simulink model "salpChain17"  (Simulink 7.8)
settings: Solver=ode15s  StartTime=0.0  StopTime=160  RelTol=1e-3
values from neighbouring files (symbols this model uses):
  angleConstraintB = 25    [15RunsSmallEtta.mat]    (also in 1To10withTorque.mat; 1To20Nodes.mat; 1To30HeadToTail.mat; 1To35FullFlip.mat)
  angleConstraintK = 400    [15RunsSmallEtta.mat]    (also in 1To10withTorque.mat; 1To20Nodes.mat; 1To30HeadToTail.mat; 1To35FullFlip.mat)
  angleLimit = 90    [15RunsSmallEtta.mat]    (also in 1To10withTorque.mat; 1To20Nodes.mat; 1To30HeadToTail.mat; 1To35FullFlip.mat)
  evenTorque = [0 0 0]    [15RunsSmallEtta.mat]    (also in 1To10withTorque.mat = [0 0 0.2]; 1To20Nodes.mat; 1To30HeadToTail.mat; 1To35FullFlip.mat)
  N = size(INPUT,1)    [SpinCalc.m]
  oddTorque = [0 0 0]    [15RunsSmallEtta.mat]    (also in 1To10withTorque.mat = [0 0 0.2]; 1To20Nodes.mat; 1To30HeadToTail.mat; 1To35FullFlip.mat)
  PropSignSw = [-1 -1 1]    [1To10withTorque.mat]    (also in 1To30HeadToTail.mat; 1To35FullFlip.mat)
  relRotInit = [0 0]    [15RunsSmallEtta.mat]    (also in 1To10withTorque.mat; 1To20Nodes.mat; 1To30HeadToTail.mat; 1To35FullFlip.mat)
  sInertia = [0.0008  0  0; 0  0.0008  0; 0  0  0.0004]    [15RunsSmallEtta.mat]    (also in 1To10withTorque.mat; 1To20Nodes.mat; 1To30HeadToTail.mat; 1To35FullFlip.mat)
  sMass = 0.04    [15RunsSmallEtta.mat]    (also in 1To10withTorque.mat; 1To20Nodes.mat; 1To30HeadToTail.mat; 1To35FullFlip.mat)
  uAmplitudeEven = [-1.03766578533 1.19688881264 1.2209450799]    [15RunsSmallEtta.mat]    (also in 1To10withTorque.mat = [-0.2 0 2]; 1To20Nodes.mat = [-0.2 0 2]; 1To30HeadToTail.mat = [-0.2 0 2]; 1To35FullFlip.mat = [-0.2 0.2 2])
libraries: mblibv1 x288
(part 5 of 5)

== system salpChain17/Salp Odd5 ==
  2DOFJointConstrainer : Subsystem
  Body : mblibv1/Bodies/Body  LConnTagsString=CS1  RConnTagsString=CG|CS5|CS4|CS2|CS3|CS6  UpdateFromCAD=off  DialogClass=MechanicalBodyBlock  Mass=sMass  MassUnits=kg  InertiaUnits=kg*m^2  Inertia=sInertia  Shape=Cylinder  ShapeDims=[1 1]  ShapeUnits=m  ShapeUse=false  Density=1  DensityUnits=kg/m^3  DensityUse=false  GraphicsMode=EQELLIPSE  BodyColorSelMode=COLORPALETTE  BodyColor=[0.16471 0.38431 0.27451]  AttachedToCS=CG  CG=Right$CG$frontConnect$CS1$CS1$m$[0 0 0]$Euler X-Y-Z$deg$CS1$true$none  WorkingFrames=Right$CS5$COPPosition$CG$CG$m$[0 0 0]$Euler X-Y-Z$deg$CS1$true$none#Right$CS4$[0 0 0]$CG$CG$m$[0 0 0]$Euler X-Y-Z$deg$CS1$true$none#Left$CS1$[0 0 0]$Adjoining$Adjoining$m$connectR$Euler X-Y-Z$deg$Adjoining$true$none#Right$CS2$backConnect$CG$CG$m$[0 0 0]$Euler X-Y-Z$deg$CS1$true$none#Right$CS3$propulsionPosition$CG$CG$m$[0 0 0]$Euler X-Y-Z$deg$CS1$true$none#Right$CS6$propulsionPosition$CG$CG$m$[0 0 0]$Euler X-Y-Z$deg$CS1$true$none  CGPos=frontConnect  CGRot=[0 0 0]  CS0Pos=[]  CS0Rot=[]  CS1Pos=[0 0 0]  CS1Rot=connectR  CS2Pos=backConnect  CS2Rot=[0 0 0]  CS3Pos=propulsionPosition  CS3Rot=[0 0 0]  CS4Pos=[0 0 0]  CS4Rot=[0 0 0]  CS5Pos=COPPosition  CS5Rot=[0 0 0]  CS6Pos=propulsionPosition  CS6Rot=[0 0 0]  CS7Pos=[]  CS7Rot=[]  CS8Pos=[]  CS8Rot=[]  CS9Pos=[]  CS9Rot=[]  CS10Pos=[]  CS10Rot=[]  CS11Pos=[]  CS11Rot=[]  CS12Pos=[]  CS12Rot=[]  CS13Pos=[]  CS13Rot=[]  CS14Pos=[]  CS14Rot=[]  CS15Pos=[]  CS15Rot=[]  CS16Pos=[]  CS16Rot=[]  CS17Pos=[]  CS17Rot=[]  CS18Pos=[]  CS18Rot=[]  CS19Pos=[]  CS19Rot=[]  CS20Pos=[]  CS20Rot=[]
  Bushing : mblibv1/Joints/Bushing  LConnTagsString=__newl0|SA1  RConnTagsString=__newr0|SA1  UpdateFromCAD=off  NumSAPorts=2  CutJoint=off  MarkAsCut=off  Primitives=prismatic_prismatic_prismatic  PrimitiveProps=P1$Follower$[1 0 0]$prismatic#P2$Follower$[0 1 0]$prismatic#P3$Follower$[0 0 1]$prismatic#R1$Follower$[1 0 0]$revolute#R2$Follower$[0 1 0]$revolute#R3$Follower$[0 0 1]$revolute  DialogClass=JointBlock  P1Axis=[1 0 0]  P2Axis=[0 1 0]  P3Axis=[0 0 1]  R1Axis=[1 0 0]  R2Axis=[0 1 0]  R3Axis=[0 0 1]
  Drag : mblibv1/Sensors &  Actuators/Body Actuator  UpdateFromCAD=off  PhysicalDomain=Mechanical  PortType=blob  ActuationStyle=Force  AngleUnits=deg  ArcVelocityUnits=deg/s  ArcAccelerationUnits=deg/s^2  CoordPositionUnits=m  VelocityUnits=m/s  AccelerationUnits=m/s^2  ForceUnits=N  TorqueUnits=N*m  ActiveIO=off  Width=6  DialogClass=MechanicalActuatorBlock  ReferenceFrame=Local (Body CS)  Angle=off  CoordPosition=on  Force=on  Torque=on
  Force Propulsion : mblibv1/Sensors &  Actuators/Body Actuator  UpdateFromCAD=off  PhysicalDomain=Mechanical  PortType=blob  ActuationStyle=Force  AngleUnits=deg  ArcVelocityUnits=deg/s  ArcAccelerationUnits=deg/s^2  CoordPositionUnits=m  VelocityUnits=m/s  AccelerationUnits=m/s^2  ForceUnits=N  TorqueUnits=N*m  ActiveIO=off  Width=3  DialogClass=MechanicalActuatorBlock  ReferenceFrame=Local (Body CS)  Angle=off  CoordPosition=on  Force=on  Torque=off
  Joint Actuator1 : mblibv1/Sensors &  Actuators/Joint Actuator  UpdateFromCAD=off  PhysicalDomain=Mechanical  PortType=blob  ActuationStyle=Force  AngleUnits=deg  ArcVelocityUnits=deg/s  ArcAccelerationUnits=deg/s^2  CoordPositionUnits=m  VelocityUnits=m/s  AccelerationUnits=m/s^2  ForceUnits=N  TorqueUnits=N*m  ActiveIO=off  Width=1  DialogClass=MechanicalActuatorBlock  Primitive=R1  ReferenceFrame=Absolute (INERTIAL)
  Joint Actuator2 : mblibv1/Sensors &  Actuators/Joint Actuator  UpdateFromCAD=off  PhysicalDomain=Mechanical  PortType=blob  ActuationStyle=Force  AngleUnits=deg  ArcVelocityUnits=deg/s  ArcAccelerationUnits=deg/s^2  CoordPositionUnits=m  VelocityUnits=m/s  AccelerationUnits=m/s^2  ForceUnits=N  TorqueUnits=N*m  ActiveIO=off  Width=1  DialogClass=MechanicalActuatorBlock  Primitive=R2  ReferenceFrame=Absolute (INERTIAL)
  Joint Initial Condition : mblibv1/Sensors &  Actuators/Joint Initial Condition  UpdateFromCAD=off  LeftPortType=blob  RightPortType=blob  PhysicalDomain=mechanical  DialogClass=InitialConditionBlock  InitialConditions=P1$false$0$m$deg$0$m/s$deg/s#P2$false$0$m$deg$0$m/s$deg/s#P3$false$0$m$deg$0$m/s$deg/s#R1$true$relRotInit(1)$m$deg$0$m/s$deg/s#R2$true$relRotInit(2)$m$deg$0$m/s$deg/s#R3$false$0$m$deg$0$m/s$deg/s#S$false$0$m$deg$0$m/s$deg/s  P1PIC=0  P1VIC=0  P2PIC=0  P2VIC=0  P3PIC=0  P3VIC=0  R1PIC=relRotInit(1)  R1VIC=0  R2PIC=relRotInit(2)  R2VIC=0  R3PIC=0  R3VIC=0  SPIC=0  SVIC=0
  Joint Spring & Damper : mblibv1/Force  Elements/Joint Spring & Damper  UpdateFromCAD=off  DialogClass=JointSpringDamper  JFEParameters=P1$true$kDrag(1)$bDrag(1)$0$m$m/s$N$deg$deg/s$N*m#P2$true$kDrag(2)$bDrag(2)$0$m$m/s$N$deg$deg/s$N*m#P3$true$kDrag(3)$bDrag(3)$0$m$m/s$N$deg$deg/s$N*m#R1$true$kDrag(4)$bDrag(4)$0$m$m/s$N$deg$deg/s$N*m#R2$true$kDrag(5)$bDrag(5)$0$m$m/s$N$deg$deg/s$N*m#R3$true$kDrag(6)$bDrag(6)$0$m$m/s$N$deg$deg/s$N*m#S$false$0$0$0$m$m/s$N$deg$deg/s$N*m
  Mechanical Branching Bar : mblibv1/Utilities/Mechanical Branching Bar  LConnTagsString=_newl0  RConnTagsString=__newr0|SA2  UpdateFromCAD=off  DialogClass=MechanicalBranchingBarBlock  NumSAPorts=2
  Mechanical Branching Bar1 : mblibv1/Utilities/Mechanical Branching Bar  LConnTagsString=_newl0  RConnTagsString=__newr0|SA2  UpdateFromCAD=off  DialogClass=MechanicalBranchingBarBlock  NumSAPorts=2
  Model : ModelReference  ModelNameDialog=v2Drag  SimulationMode=Normal  ModelReferenceVersion=1.20  CopyOfModelName=v2Drag  DefaultDataLogging=on
  Mux : Mux  Inputs=2
  Torque Propulsion : mblibv1/Sensors &  Actuators/Body Actuator  UpdateFromCAD=off  PhysicalDomain=Mechanical  PortType=blob  ActuationStyle=Force  AngleUnits=deg  ArcVelocityUnits=deg/s  ArcAccelerationUnits=deg/s^2  CoordPositionUnits=m  VelocityUnits=m/s  AccelerationUnits=m/s^2  ForceUnits=N  TorqueUnits=N*m  ActiveIO=off  Width=3  DialogClass=MechanicalActuatorBlock  ReferenceFrame=Local (Body CS)  Angle=off  CoordPosition=on  Force=off  Torque=on
  Universal : mblibv1/Joints/Universal  LConnTagsString=__newl0|SA1|SA2  RConnTagsString=__newr0|SA1|SA2  UpdateFromCAD=off  NumSAPorts=4  CutJoint=off  MarkAsCut=off  Primitives=prismatic  PrimitiveProps=R1$Base$u1axis$revolute#R2$Base$u2axis$revolute  DialogClass=JointBlock  R1Axis=u1axis  R2Axis=u2axis
  angle 2 : mblibv1/Sensors &  Actuators/Joint Sensor  UpdateFromCAD=off  PhysicalDomain=Mechanical  PortType=blob  Muxed=on  Pose=off  Angle=on  AngleUnits=deg  ArcVelocity=off  ArcVelocityUnits=deg/s  ArcAcceleration=off  ArcAccelerationUnits=deg/s^2  CoordPosition=on  CoordPositionUnits=m  Velocity=off  VelocityUnits=m/s  Acceleration=off  AccelerationUnits=m/s^2  Quaternion=on  QuaternionDT=off  QuaternionDDT=off  QuaternionUnits=off  OutputVector=[1]  ActiveIO=off  Width=1  DialogClass=MechanicalSensorBlock  Primitive=R2  Force=off  ForceUnits=N  Torque=off  TorqueUnits=N*m  ReferenceFrame=Absolute (World)  ReactionSensedSide=Base  ReactionReferenceFrame=Absolute (World)  ReactionForce=off  ReactionForceUnits=N  ReactionMoment=off  ReactionMomentUnits=N*m
  angle1 : mblibv1/Sensors &  Actuators/Joint Sensor  UpdateFromCAD=off  PhysicalDomain=Mechanical  PortType=blob  Muxed=on  Pose=off  Angle=on  AngleUnits=deg  ArcVelocity=off  ArcVelocityUnits=deg/s  ArcAcceleration=off  ArcAccelerationUnits=deg/s^2  CoordPosition=on  CoordPositionUnits=m  Velocity=off  VelocityUnits=m/s  Acceleration=off  AccelerationUnits=m/s^2  Quaternion=on  QuaternionDT=off  QuaternionDDT=off  QuaternionUnits=off  OutputVector=[1]  ActiveIO=off  Width=1  DialogClass=MechanicalSensorBlock  Primitive=R1  Force=off  ForceUnits=N  Torque=off  TorqueUnits=N*m  ReferenceFrame=Absolute (World)  ReactionSensedSide=Base  ReactionReferenceFrame=Absolute (World)  ReactionForce=off  ReactionForceUnits=N  ReactionMoment=off  ReactionMomentUnits=N*m
  angular velocity body frame : mblibv1/Sensors &  Actuators/Body Sensor  UpdateFromCAD=off  PhysicalDomain=Mechanical  PortType=blob  Muxed=off  Pose=off  Angle=on  AngleUnits=deg  ArcVelocity=on  ArcVelocityUnits=deg/s  ArcAcceleration=off  ArcAccelerationUnits=deg/s^2  CoordPosition=off  CoordPositionUnits=m  Velocity=off  VelocityUnits=m/s  Acceleration=off  AccelerationUnits=m/s^2  Quaternion=on  QuaternionDT=off  QuaternionDDT=off  QuaternionUnits=off  OutputVector=[1]  ActiveIO=off  Width=3  DialogClass=MechanicalSensorBlock  ReferenceFrame=Local (Body CS)
  dummy body for drag : mblibv1/Bodies/Body  LConnTagsString=CS1  RConnTagsString=CS2  UpdateFromCAD=off  DialogClass=MechanicalBodyBlock  Mass=sMass/100  MassUnits=kg  InertiaUnits=kg*m^2  Inertia=eye(3)/1000  Shape=Cylinder  ShapeDims=[1 1]  ShapeUnits=m  ShapeUse=false  Density=1  DensityUnits=kg/m^3  DensityUse=false  GraphicsMode=CONVHULL  BodyColorSelMode=COLORPALETTE  BodyColor=[1 0 1]  AttachedToCS=CG  CG=Left$CG$[0 0 0]$CS1$CS1$m$[0 0 0]$Euler X-Y-Z$deg$CS1$false$none  WorkingFrames=Left$CS1$[0 0 0]$Adjoining$Adjoining$m$[0 0 0]$Euler X-Y-Z$deg$Adjoining$true$none#Right$CS2$[0 0 0]$CS1$CS1$m$[0 0 0]$Euler X-Y-Z$deg$CS1$true$none  CGPos=[0 0 0]  CGRot=[0 0 0]  CS0Pos=[]  CS0Rot=[]  CS1Pos=[0 0 0]  CS1Rot=[0 0 0]  CS2Pos=[0 0 0]  CS2Rot=[0 0 0]  CS3Pos=[]  CS3Rot=[]  CS4Pos=[]  CS4Rot=[]  CS5Pos=[]  CS5Rot=[]  CS6Pos=[]  CS6Rot=[]  CS7Pos=[]  CS7Rot=[]  CS8Pos=[]  CS8Rot=[]  CS9Pos=[]  CS9Rot=[]  CS10Pos=[]  CS10Rot=[]  CS11Pos=[]  CS11Rot=[]  CS12Pos=[]  CS12Rot=[]  CS13Pos=[]  CS13Rot=[]  CS14Pos=[]  CS14Rot=[]  CS15Pos=[]  CS15Rot=[]  CS16Pos=[]  CS16Rot=[]  CS17Pos=[]  CS17Rot=[]  CS18Pos=[]  CS18Rot=[]  CS19Pos=[]  CS19Rot=[]  CS20Pos=[]  CS20Rot=[]
  translation body frame : mblibv1/Sensors &  Actuators/Body Sensor  UpdateFromCAD=off  PhysicalDomain=Mechanical  PortType=blob  Muxed=off  Pose=off  Angle=on  AngleUnits=deg  ArcVelocity=off  ArcVelocityUnits=deg/s  ArcAcceleration=off  ArcAccelerationUnits=deg/s^2  CoordPosition=off  CoordPositionUnits=m  Velocity=on  VelocityUnits=m/s  Acceleration=off  AccelerationUnits=m/s^2  Quaternion=on  QuaternionDT=off  QuaternionDDT=off  QuaternionUnits=off  OutputVector=[1]  ActiveIO=off  Width=3  DialogClass=MechanicalSensorBlock  ReferenceFrame=Local (Body CS)
  Front : PMIOPort  Port=1  Side=Left
  Back : PMIOPort  Port=2  Side=Right
  wires:
  translation body frame/1 -> Model/1
  Mux/1 -> Drag/1
  angular velocity body frame/1 -> Model/2
  angle 2/1 -> 2DOFJointConstrainer/2(In2)  "angle2"
  angle1/1 -> 2DOFJointConstrainer/1(In1)  "angle1"
  Model/1 -> Mux/1
  Model/2 -> Mux/2
  [OddAmplitude] -> Force Propulsion/1
  [OddTorque] -> Torque Propulsion/1
  2DOFJointConstrainer/1(Out1) -> Joint Actuator1/1
  2DOFJointConstrainer/2(Out2) -> Joint Actuator2/1
  connections:
  Body/RConn3 -- Mechanical Branching Bar/LConn1
  dummy body for drag/RConn1 -- Drag/RConn1
  Mechanical Branching Bar/RConn1 -- angular velocity body frame/LConn1
  translation body frame/LConn1 -- Mechanical Branching Bar/RConn2
  Bushing/RConn1 -- Body/RConn2
  Bushing/LConn1 -- dummy body for drag/LConn1
  Bushing/RConn2 -- Joint Spring & Damper/LConn1
  Front/RConn1 -- Body/LConn1
  Universal/RConn1 -- Back/RConn1
  Universal/LConn1 -- Body/RConn4
  Universal/LConn2 -- Joint Initial Condition/RConn1
  Force Propulsion/RConn1 -- Body/RConn5
  Universal/RConn2 -- Mechanical Branching Bar1/LConn1
  Mechanical Branching Bar1/RConn1 -- angle1/LConn1
  Mechanical Branching Bar1/RConn2 -- angle 2/LConn1
  Torque Propulsion/RConn1 -- Body/RConn6
  Universal/RConn3 -- Joint Actuator1/RConn1
  Joint Actuator2/RConn1 -- Universal/LConn3

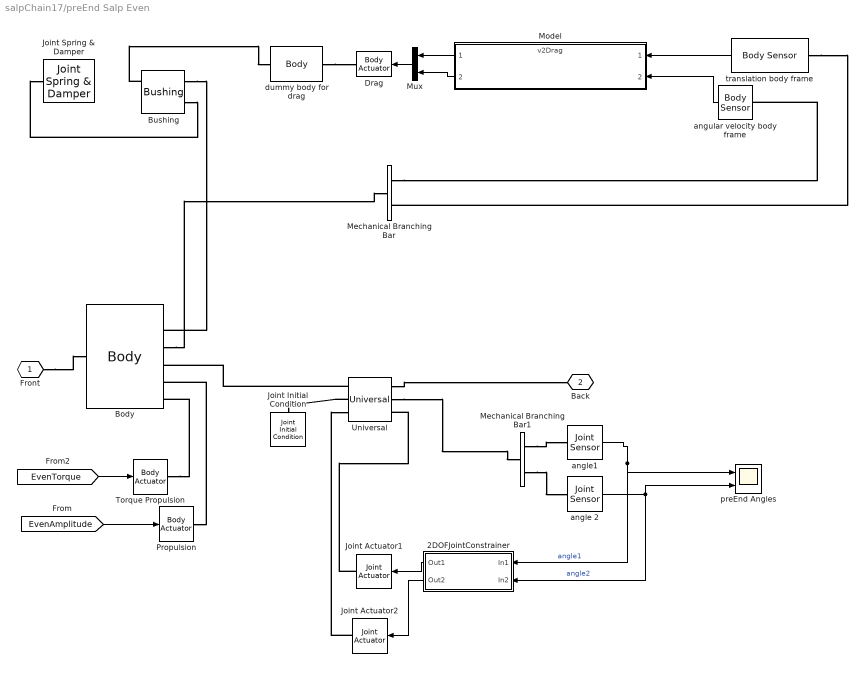
== system salpChain17/preEnd Salp Even ==
  2DOFJointConstrainer : Subsystem
  Body : mblibv1/Bodies/Body  LConnTagsString=CS1  RConnTagsString=CG|CS5|CS4|CS2|CS3|CS6  UpdateFromCAD=off  DialogClass=MechanicalBodyBlock  Mass=sMass  MassUnits=kg  InertiaUnits=kg*m^2  Inertia=sInertia  Shape=Cylinder  ShapeDims=[1 1]  ShapeUnits=m  ShapeUse=false  Density=1  DensityUnits=kg/m^3  DensityUse=false  GraphicsMode=EQELLIPSE  BodyColorSelMode=COLORPALETTE  BodyColor=[0.16471 0.38431 0.27451]  AttachedToCS=CG  CG=Right$CG$frontConnect$CS1$CS1$m$[0 0 0]$Euler X-Y-Z$deg$CS1$true$none  WorkingFrames=Right$CS5$COPPosition$CG$CG$m$[0 0 0]$Euler X-Y-Z$deg$CS1$true$none#Right$CS4$[0 0 0]$CG$CG$m$[0 0 0]$Euler X-Y-Z$deg$CS1$true$none#Left$CS1$[0 0 0]$Adjoining$Adjoining$m$connectR$Euler X-Y-Z$deg$Adjoining$true$none#Right$CS2$backConnect$CG$CG$m$[0 0 0]$Euler X-Y-Z$deg$CS1$true$none#Right$CS3$propulsionPosition$CG$CG$m$[0 0 0]$Euler X-Y-Z$deg$CS1$true$none#Right$CS6$propulsionPosition$CG$CG$m$[0 0 0]$Euler X-Y-Z$deg$CS1$true$none  CGPos=frontConnect  CGRot=[0 0 0]  CS0Pos=[]  CS0Rot=[]  CS1Pos=[0 0 0]  CS1Rot=connectR  CS2Pos=backConnect  CS2Rot=[0 0 0]  CS3Pos=propulsionPosition  CS3Rot=[0 0 0]  CS4Pos=[0 0 0]  CS4Rot=[0 0 0]  CS5Pos=COPPosition  CS5Rot=[0 0 0]  CS6Pos=propulsionPosition  CS6Rot=[0 0 0]  CS7Pos=[]  CS7Rot=[]  CS8Pos=[]  CS8Rot=[]  CS9Pos=[]  CS9Rot=[]  CS10Pos=[]  CS10Rot=[]  CS11Pos=[]  CS11Rot=[]  CS12Pos=[]  CS12Rot=[]  CS13Pos=[]  CS13Rot=[]  CS14Pos=[]  CS14Rot=[]  CS15Pos=[]  CS15Rot=[]  CS16Pos=[]  CS16Rot=[]  CS17Pos=[]  CS17Rot=[]  CS18Pos=[]  CS18Rot=[]  CS19Pos=[]  CS19Rot=[]  CS20Pos=[]  CS20Rot=[]
  Bushing : mblibv1/Joints/Bushing  LConnTagsString=__newl0|SA1  RConnTagsString=__newr0|SA1  UpdateFromCAD=off  NumSAPorts=2  CutJoint=off  MarkAsCut=off  Primitives=prismatic_prismatic_prismatic  PrimitiveProps=P1$Follower$[1 0 0]$prismatic#P2$Follower$[0 1 0]$prismatic#P3$Follower$[0 0 1]$prismatic#R1$Follower$[1 0 0]$revolute#R2$Follower$[0 1 0]$revolute#R3$Follower$[0 0 1]$revolute  DialogClass=JointBlock  P1Axis=[1 0 0]  P2Axis=[0 1 0]  P3Axis=[0 0 1]  R1Axis=[1 0 0]  R2Axis=[0 1 0]  R3Axis=[0 0 1]
  Drag : mblibv1/Sensors &  Actuators/Body Actuator  UpdateFromCAD=off  PhysicalDomain=Mechanical  PortType=blob  ActuationStyle=Force  AngleUnits=deg  ArcVelocityUnits=deg/s  ArcAccelerationUnits=deg/s^2  CoordPositionUnits=m  VelocityUnits=m/s  AccelerationUnits=m/s^2  ForceUnits=N  TorqueUnits=N*m  ActiveIO=off  Width=6  DialogClass=MechanicalActuatorBlock  ReferenceFrame=Local (Body CS)  Angle=off  CoordPosition=on  Force=on  Torque=on
  Joint Actuator1 : mblibv1/Sensors &  Actuators/Joint Actuator  UpdateFromCAD=off  PhysicalDomain=Mechanical  PortType=blob  ActuationStyle=Force  AngleUnits=deg  ArcVelocityUnits=deg/s  ArcAccelerationUnits=deg/s^2  CoordPositionUnits=m  VelocityUnits=m/s  AccelerationUnits=m/s^2  ForceUnits=N  TorqueUnits=N*m  ActiveIO=off  Width=1  DialogClass=MechanicalActuatorBlock  Primitive=R1  ReferenceFrame=Absolute (INERTIAL)
  Joint Actuator2 : mblibv1/Sensors &  Actuators/Joint Actuator  UpdateFromCAD=off  PhysicalDomain=Mechanical  PortType=blob  ActuationStyle=Force  AngleUnits=deg  ArcVelocityUnits=deg/s  ArcAccelerationUnits=deg/s^2  CoordPositionUnits=m  VelocityUnits=m/s  AccelerationUnits=m/s^2  ForceUnits=N  TorqueUnits=N*m  ActiveIO=off  Width=1  DialogClass=MechanicalActuatorBlock  Primitive=R2  ReferenceFrame=Absolute (INERTIAL)
  Joint Initial Condition : mblibv1/Sensors &  Actuators/Joint Initial Condition  UpdateFromCAD=off  LeftPortType=blob  RightPortType=blob  PhysicalDomain=mechanical  DialogClass=InitialConditionBlock  InitialConditions=P1$false$0$m$deg$0$m/s$deg/s#P2$false$0$m$deg$0$m/s$deg/s#P3$false$0$m$deg$0$m/s$deg/s#R1$true$relRotInit(1)$m$deg$0$m/s$deg/s#R2$true$relRotInit(2)$m$deg$0$m/s$deg/s#R3$false$0$m$deg$0$m/s$deg/s#S$false$0$m$deg$0$m/s$deg/s  P1PIC=0  P1VIC=0  P2PIC=0  P2VIC=0  P3PIC=0  P3VIC=0  R1PIC=relRotInit(1)  R1VIC=0  R2PIC=relRotInit(2)  R2VIC=0  R3PIC=0  R3VIC=0  SPIC=0  SVIC=0
  Joint Spring & Damper : mblibv1/Force  Elements/Joint Spring & Damper  UpdateFromCAD=off  DialogClass=JointSpringDamper  JFEParameters=P1$true$kDrag(1)$bDrag(1)$0$m$m/s$N$deg$deg/s$N*m#P2$true$kDrag(2)$bDrag(2)$0$m$m/s$N$deg$deg/s$N*m#P3$true$kDrag(3)$bDrag(3)$0$m$m/s$N$deg$deg/s$N*m#R1$true$kDrag(4)$bDrag(4)$0$m$m/s$N$deg$deg/s$N*m#R2$true$kDrag(5)$bDrag(5)$0$m$m/s$N$deg$deg/s$N*m#R3$true$kDrag(6)$bDrag(6)$0$m$m/s$N$deg$deg/s$N*m#S$false$0$0$0$m$m/s$N$deg$deg/s$N*m
  Mechanical Branching Bar : mblibv1/Utilities/Mechanical Branching Bar  LConnTagsString=_newl0  RConnTagsString=__newr0|SA2  UpdateFromCAD=off  DialogClass=MechanicalBranchingBarBlock  NumSAPorts=2
  Mechanical Branching Bar1 : mblibv1/Utilities/Mechanical Branching Bar  LConnTagsString=_newl0  RConnTagsString=__newr0|SA2  UpdateFromCAD=off  DialogClass=MechanicalBranchingBarBlock  NumSAPorts=2
  Model : ModelReference  ModelNameDialog=v2Drag  SimulationMode=Normal  ModelReferenceVersion=1.20  CopyOfModelName=v2Drag  DefaultDataLogging=on
  Mux : Mux  Inputs=2
  Propulsion : mblibv1/Sensors &  Actuators/Body Actuator  UpdateFromCAD=off  PhysicalDomain=Mechanical  PortType=blob  ActuationStyle=Force  AngleUnits=deg  ArcVelocityUnits=deg/s  ArcAccelerationUnits=deg/s^2  CoordPositionUnits=m  VelocityUnits=m/s  AccelerationUnits=m/s^2  ForceUnits=N  TorqueUnits=N*m  ActiveIO=off  Width=3  DialogClass=MechanicalActuatorBlock  ReferenceFrame=Local (Body CS)  Angle=off  CoordPosition=on  Force=on  Torque=off
  Torque Propulsion : mblibv1/Sensors &  Actuators/Body Actuator  UpdateFromCAD=off  PhysicalDomain=Mechanical  PortType=blob  ActuationStyle=Force  AngleUnits=deg  ArcVelocityUnits=deg/s  ArcAccelerationUnits=deg/s^2  CoordPositionUnits=m  VelocityUnits=m/s  AccelerationUnits=m/s^2  ForceUnits=N  TorqueUnits=N*m  ActiveIO=off  Width=3  DialogClass=MechanicalActuatorBlock  ReferenceFrame=Local (Body CS)  Angle=off  CoordPosition=on  Force=off  Torque=on
  Universal : mblibv1/Joints/Universal  LConnTagsString=__newl0|SA1|SA2  RConnTagsString=__newr0|SA1|SA2  UpdateFromCAD=off  NumSAPorts=4  CutJoint=off  MarkAsCut=off  Primitives=prismatic  PrimitiveProps=R1$Base$u1axis$revolute#R2$Base$u2axis$revolute  DialogClass=JointBlock  R1Axis=u1axis  R2Axis=u2axis
  angle 2 : mblibv1/Sensors &  Actuators/Joint Sensor  UpdateFromCAD=off  PhysicalDomain=Mechanical  PortType=blob  Muxed=on  Pose=off  Angle=on  AngleUnits=deg  ArcVelocity=off  ArcVelocityUnits=deg/s  ArcAcceleration=off  ArcAccelerationUnits=deg/s^2  CoordPosition=on  CoordPositionUnits=m  Velocity=off  VelocityUnits=m/s  Acceleration=off  AccelerationUnits=m/s^2  Quaternion=on  QuaternionDT=off  QuaternionDDT=off  QuaternionUnits=off  OutputVector=[1]  ActiveIO=off  Width=1  DialogClass=MechanicalSensorBlock  Primitive=R2  Force=off  ForceUnits=N  Torque=off  TorqueUnits=N*m  ReferenceFrame=Absolute (World)  ReactionSensedSide=Base  ReactionReferenceFrame=Absolute (World)  ReactionForce=off  ReactionForceUnits=N  ReactionMoment=off  ReactionMomentUnits=N*m
  angle1 : mblibv1/Sensors &  Actuators/Joint Sensor  UpdateFromCAD=off  PhysicalDomain=Mechanical  PortType=blob  Muxed=on  Pose=off  Angle=on  AngleUnits=deg  ArcVelocity=off  ArcVelocityUnits=deg/s  ArcAcceleration=off  ArcAccelerationUnits=deg/s^2  CoordPosition=on  CoordPositionUnits=m  Velocity=off  VelocityUnits=m/s  Acceleration=off  AccelerationUnits=m/s^2  Quaternion=on  QuaternionDT=off  QuaternionDDT=off  QuaternionUnits=off  OutputVector=[1]  ActiveIO=off  Width=1  DialogClass=MechanicalSensorBlock  Primitive=R1  Force=off  ForceUnits=N  Torque=off  TorqueUnits=N*m  ReferenceFrame=Absolute (World)  ReactionSensedSide=Base  ReactionReferenceFrame=Absolute (World)  ReactionForce=off  ReactionForceUnits=N  ReactionMoment=off  ReactionMomentUnits=N*m
  angular velocity body frame : mblibv1/Sensors &  Actuators/Body Sensor  UpdateFromCAD=off  PhysicalDomain=Mechanical  PortType=blob  Muxed=off  Pose=off  Angle=on  AngleUnits=deg  ArcVelocity=on  ArcVelocityUnits=deg/s  ArcAcceleration=off  ArcAccelerationUnits=deg/s^2  CoordPosition=off  CoordPositionUnits=m  Velocity=off  VelocityUnits=m/s  Acceleration=off  AccelerationUnits=m/s^2  Quaternion=on  QuaternionDT=off  QuaternionDDT=off  QuaternionUnits=off  OutputVector=[1]  ActiveIO=off  Width=3  DialogClass=MechanicalSensorBlock  ReferenceFrame=Local (Body CS)
  dummy body for drag : mblibv1/Bodies/Body  LConnTagsString=CS1  RConnTagsString=CS2  UpdateFromCAD=off  DialogClass=MechanicalBodyBlock  Mass=sMass/100  MassUnits=kg  InertiaUnits=kg*m^2  Inertia=eye(3)/1000  Shape=Cylinder  ShapeDims=[1 1]  ShapeUnits=m  ShapeUse=false  Density=1  DensityUnits=kg/m^3  DensityUse=false  GraphicsMode=CONVHULL  BodyColorSelMode=COLORPALETTE  BodyColor=[1 0 1]  AttachedToCS=CG  CG=Left$CG$[0 0 0]$CS1$CS1$m$[0 0 0]$Euler X-Y-Z$deg$CS1$false$none  WorkingFrames=Left$CS1$[0 0 0]$Adjoining$Adjoining$m$[0 0 0]$Euler X-Y-Z$deg$Adjoining$true$none#Right$CS2$[0 0 0]$CS1$CS1$m$[0 0 0]$Euler X-Y-Z$deg$CS1$true$none  CGPos=[0 0 0]  CGRot=[0 0 0]  CS0Pos=[]  CS0Rot=[]  CS1Pos=[0 0 0]  CS1Rot=[0 0 0]  CS2Pos=[0 0 0]  CS2Rot=[0 0 0]  CS3Pos=[]  CS3Rot=[]  CS4Pos=[]  CS4Rot=[]  CS5Pos=[]  CS5Rot=[]  CS6Pos=[]  CS6Rot=[]  CS7Pos=[]  CS7Rot=[]  CS8Pos=[]  CS8Rot=[]  CS9Pos=[]  CS9Rot=[]  CS10Pos=[]  CS10Rot=[]  CS11Pos=[]  CS11Rot=[]  CS12Pos=[]  CS12Rot=[]  CS13Pos=[]  CS13Rot=[]  CS14Pos=[]  CS14Rot=[]  CS15Pos=[]  CS15Rot=[]  CS16Pos=[]  CS16Rot=[]  CS17Pos=[]  CS17Rot=[]  CS18Pos=[]  CS18Rot=[]  CS19Pos=[]  CS19Rot=[]  CS20Pos=[]  CS20Rot=[]
  preEnd Angles : Scope  NumInputPorts=2
      settings: YMin=-40~0  YMax=5~60  SaveName=preEndSalp_angles  MaxDataPoints=9000
  translation body frame : mblibv1/Sensors &  Actuators/Body Sensor  UpdateFromCAD=off  PhysicalDomain=Mechanical  PortType=blob  Muxed=off  Pose=off  Angle=on  AngleUnits=deg  ArcVelocity=off  ArcVelocityUnits=deg/s  ArcAcceleration=off  ArcAccelerationUnits=deg/s^2  CoordPosition=off  CoordPositionUnits=m  Velocity=on  VelocityUnits=m/s  Acceleration=off  AccelerationUnits=m/s^2  Quaternion=on  QuaternionDT=off  QuaternionDDT=off  QuaternionUnits=off  OutputVector=[1]  ActiveIO=off  Width=3  DialogClass=MechanicalSensorBlock  ReferenceFrame=Local (Body CS)
  Front : PMIOPort  Port=1  Side=Left
  Back : PMIOPort  Port=2  Side=Right
  wires:
  translation body frame/1 -> Model/1
  Mux/1 -> Drag/1
  angular velocity body frame/1 -> Model/2
  angle 2/1 -> 2DOFJointConstrainer/2(In2), preEnd Angles/2  "angle2"
  angle1/1 -> 2DOFJointConstrainer/1(In1), preEnd Angles/1  "angle1"
  Model/1 -> Mux/1
  Model/2 -> Mux/2
  [EvenAmplitude] -> Propulsion/1
  [EvenTorque] -> Torque Propulsion/1
  2DOFJointConstrainer/1(Out1) -> Joint Actuator1/1
  2DOFJointConstrainer/2(Out2) -> Joint Actuator2/1
  connections:
  Body/RConn3 -- Mechanical Branching Bar/LConn1
  dummy body for drag/RConn1 -- Drag/RConn1
  Mechanical Branching Bar/RConn1 -- angular velocity body frame/LConn1
  translation body frame/LConn1 -- Mechanical Branching Bar/RConn2
  Bushing/RConn1 -- Body/RConn2
  Bushing/LConn1 -- dummy body for drag/LConn1
  Bushing/RConn2 -- Joint Spring & Damper/LConn1
  Front/RConn1 -- Body/LConn1
  Universal/RConn1 -- Back/RConn1
  Universal/LConn1 -- Body/RConn4
  Universal/LConn2 -- Joint Initial Condition/RConn1
  Propulsion/RConn1 -- Body/RConn5
  Universal/RConn2 -- Mechanical Branching Bar1/LConn1
  Mechanical Branching Bar1/RConn1 -- angle1/LConn1
  Mechanical Branching Bar1/RConn2 -- angle 2/LConn1
  Torque Propulsion/RConn1 -- Body/RConn6
  Joint Actuator1/RConn1 -- Universal/RConn3
  Joint Actuator2/RConn1 -- Universal/LConn3

== system salpChain17/First Salp Odd/2DOFJointConstrainer ==
  In1 : Inport
  In2 : Inport  Port=2
  AnglleConstrainer1 : Subsystem
  AnglleConstrainer2 : Subsystem
  Out1 : Outport
  Out2 : Outport  Port=2
  wires:
  In1/1 -> AnglleConstrainer1/1(In1)
  AnglleConstrainer1/1(Out1) -> Out1/1
  In2/1 -> AnglleConstrainer2/1(In1)
  AnglleConstrainer2/1(Out1) -> Out2/1

== system salpChain17/Middle Salp Odd/2DOFJointConstrainer ==
  In1 : Inport
  In2 : Inport  Port=2
  AnglleConstrainer1 : Subsystem
  AnglleConstrainer2 : Subsystem
  Out1 : Outport
  Out2 : Outport  Port=2
  wires:
  In1/1 -> AnglleConstrainer1/1(In1)
  AnglleConstrainer1/1(Out1) -> Out1/1
  In2/1 -> AnglleConstrainer2/1(In1)
  AnglleConstrainer2/1(Out1) -> Out2/1

== system salpChain17/Salp Even/2DOFJointConstrainer ==
  In1 : Inport
  In2 : Inport  Port=2
  AnglleConstrainer1 : Subsystem
  AnglleConstrainer2 : Subsystem
  Out1 : Outport
  Out2 : Outport  Port=2
  wires:
  In1/1 -> AnglleConstrainer1/1(In1)
  AnglleConstrainer1/1(Out1) -> Out1/1
  In2/1 -> AnglleConstrainer2/1(In1)
  AnglleConstrainer2/1(Out1) -> Out2/1

== system salpChain17/Salp Even1/2DOFJointConstrainer ==
  In1 : Inport
  In2 : Inport  Port=2
  AnglleConstrainer1 : Subsystem
  AnglleConstrainer2 : Subsystem
  Out1 : Outport
  Out2 : Outport  Port=2
  wires:
  In1/1 -> AnglleConstrainer1/1(In1)
  AnglleConstrainer1/1(Out1) -> Out1/1
  In2/1 -> AnglleConstrainer2/1(In1)
  AnglleConstrainer2/1(Out1) -> Out2/1

== system salpChain17/Salp Even2/2DOFJointConstrainer ==
  In1 : Inport
  In2 : Inport  Port=2
  AnglleConstrainer1 : Subsystem
  AnglleConstrainer2 : Subsystem
  Out1 : Outport
  Out2 : Outport  Port=2
  wires:
  In1/1 -> AnglleConstrainer1/1(In1)
  AnglleConstrainer1/1(Out1) -> Out1/1
  In2/1 -> AnglleConstrainer2/1(In1)
  AnglleConstrainer2/1(Out1) -> Out2/1

== system salpChain17/Salp Even3/2DOFJointConstrainer ==
  In1 : Inport
  In2 : Inport  Port=2
  AnglleConstrainer1 : Subsystem
  AnglleConstrainer2 : Subsystem
  Out1 : Outport
  Out2 : Outport  Port=2
  wires:
  In1/1 -> AnglleConstrainer1/1(In1)
  AnglleConstrainer1/1(Out1) -> Out1/1
  In2/1 -> AnglleConstrainer2/1(In1)
  AnglleConstrainer2/1(Out1) -> Out2/1

== system salpChain17/Salp Even4/2DOFJointConstrainer ==
  In1 : Inport
  In2 : Inport  Port=2
  AnglleConstrainer1 : Subsystem
  AnglleConstrainer2 : Subsystem
  Out1 : Outport
  Out2 : Outport  Port=2
  wires:
  In1/1 -> AnglleConstrainer1/1(In1)
  AnglleConstrainer1/1(Out1) -> Out1/1
  In2/1 -> AnglleConstrainer2/1(In1)
  AnglleConstrainer2/1(Out1) -> Out2/1

== system salpChain17/Salp Even5/2DOFJointConstrainer ==
  In1 : Inport
  In2 : Inport  Port=2
  AnglleConstrainer1 : Subsystem
  AnglleConstrainer2 : Subsystem
  Out1 : Outport
  Out2 : Outport  Port=2
  wires:
  In1/1 -> AnglleConstrainer1/1(In1)
  AnglleConstrainer1/1(Out1) -> Out1/1
  In2/1 -> AnglleConstrainer2/1(In1)
  AnglleConstrainer2/1(Out1) -> Out2/1

== system salpChain17/Salp Even6/2DOFJointConstrainer ==
  In1 : Inport
  In2 : Inport  Port=2
  AnglleConstrainer1 : Subsystem
  AnglleConstrainer2 : Subsystem
  Out1 : Outport
  Out2 : Outport  Port=2
  wires:
  In1/1 -> AnglleConstrainer1/1(In1)
  AnglleConstrainer1/1(Out1) -> Out1/1
  In2/1 -> AnglleConstrainer2/1(In1)
  AnglleConstrainer2/1(Out1) -> Out2/1

== system salpChain17/Salp Odd/2DOFJointConstrainer ==
  In1 : Inport
  In2 : Inport  Port=2
  AnglleConstrainer1 : Subsystem
  AnglleConstrainer2 : Subsystem
  Out1 : Outport
  Out2 : Outport  Port=2
  wires:
  In1/1 -> AnglleConstrainer1/1(In1)
  AnglleConstrainer1/1(Out1) -> Out1/1
  In2/1 -> AnglleConstrainer2/1(In1)
  AnglleConstrainer2/1(Out1) -> Out2/1

== system salpChain17/Salp Odd1/2DOFJointConstrainer ==
  In1 : Inport
  In2 : Inport  Port=2
  AnglleConstrainer1 : Subsystem
  AnglleConstrainer2 : Subsystem
  Out1 : Outport
  Out2 : Outport  Port=2
  wires:
  In1/1 -> AnglleConstrainer1/1(In1)
  AnglleConstrainer1/1(Out1) -> Out1/1
  In2/1 -> AnglleConstrainer2/1(In1)
  AnglleConstrainer2/1(Out1) -> Out2/1

== system salpChain17/Salp Odd2/2DOFJointConstrainer ==
  In1 : Inport
  In2 : Inport  Port=2
  AnglleConstrainer1 : Subsystem
  AnglleConstrainer2 : Subsystem
  Out1 : Outport
  Out2 : Outport  Port=2
  wires:
  In1/1 -> AnglleConstrainer1/1(In1)
  AnglleConstrainer1/1(Out1) -> Out1/1
  In2/1 -> AnglleConstrainer2/1(In1)
  AnglleConstrainer2/1(Out1) -> Out2/1

== system salpChain17/Salp Odd3/2DOFJointConstrainer ==
  In1 : Inport
  In2 : Inport  Port=2
  AnglleConstrainer1 : Subsystem
  AnglleConstrainer2 : Subsystem
  Out1 : Outport
  Out2 : Outport  Port=2
  wires:
  In1/1 -> AnglleConstrainer1/1(In1)
  AnglleConstrainer1/1(Out1) -> Out1/1
  In2/1 -> AnglleConstrainer2/1(In1)
  AnglleConstrainer2/1(Out1) -> Out2/1

== system salpChain17/Salp Odd4/2DOFJointConstrainer ==
  In1 : Inport
  In2 : Inport  Port=2
  AnglleConstrainer1 : Subsystem
  AnglleConstrainer2 : Subsystem
  Out1 : Outport
  Out2 : Outport  Port=2
  wires:
  In1/1 -> AnglleConstrainer1/1(In1)
  AnglleConstrainer1/1(Out1) -> Out1/1
  In2/1 -> AnglleConstrainer2/1(In1)
  AnglleConstrainer2/1(Out1) -> Out2/1

== system salpChain17/Salp Odd5/2DOFJointConstrainer ==
  In1 : Inport
  In2 : Inport  Port=2
  AnglleConstrainer1 : Subsystem
  AnglleConstrainer2 : Subsystem
  Out1 : Outport
  Out2 : Outport  Port=2
  wires:
  In1/1 -> AnglleConstrainer1/1(In1)
  AnglleConstrainer1/1(Out1) -> Out1/1
  In2/1 -> AnglleConstrainer2/1(In1)
  AnglleConstrainer2/1(Out1) -> Out2/1

== system salpChain17/preEnd Salp Even/2DOFJointConstrainer ==
  In1 : Inport
  In2 : Inport  Port=2
  AnglleConstrainer1 : Subsystem
  AnglleConstrainer2 : Subsystem
  Out1 : Outport
  Out2 : Outport  Port=2
  wires:
  In1/1 -> AnglleConstrainer1/1(In1)
  AnglleConstrainer1/1(Out1) -> Out1/1
  In2/1 -> AnglleConstrainer2/1(In1)
  AnglleConstrainer2/1(Out1) -> Out2/1

== system salpChain17/First Salp Odd/2DOFJointConstrainer/AnglleConstrainer1 ==
  In1 : Inport
  Dead Zone : DeadZone  LowerValue=-angleLimit  UpperValue=angleLimit  LinearizeAsGain=off  SaturateOnIntegerOverflow=on
  Derivative : Derivative
  P : Gain  Gain=-angleConstraintK
  P1 : Gain  Gain=-angleConstraintB
  Sum : Sum  Inputs=|++
  Out1 : Outport
  wires:
  Derivative/1 -> P1/1
  P1/1 -> Sum/2
  P/1 -> Sum/1
  Sum/1 -> Out1/1
  In1/1 -> Dead Zone/1
  Dead Zone/1 -> P/1, Derivative/1

== system salpChain17/First Salp Odd/2DOFJointConstrainer/AnglleConstrainer2 ==
  In1 : Inport
  Dead Zone : DeadZone  LowerValue=-angleLimit  UpperValue=angleLimit  LinearizeAsGain=off  SaturateOnIntegerOverflow=on
  Derivative : Derivative
  P : Gain  Gain=-angleConstraintK
  P1 : Gain  Gain=-angleConstraintB
  Sum : Sum  Inputs=|++
  Out1 : Outport
  wires:
  Derivative/1 -> P1/1
  P1/1 -> Sum/2
  P/1 -> Sum/1
  Sum/1 -> Out1/1
  In1/1 -> Dead Zone/1
  Dead Zone/1 -> P/1, Derivative/1

== system salpChain17/Middle Salp Odd/2DOFJointConstrainer/AnglleConstrainer1 ==
  In1 : Inport
  Dead Zone : DeadZone  LowerValue=-angleLimit  UpperValue=angleLimit  LinearizeAsGain=off  SaturateOnIntegerOverflow=on
  Derivative : Derivative
  P : Gain  Gain=-angleConstraintK
  P1 : Gain  Gain=-angleConstraintB
  Sum : Sum  Inputs=|++
  Out1 : Outport
  wires:
  Derivative/1 -> P1/1
  P1/1 -> Sum/2
  P/1 -> Sum/1
  Sum/1 -> Out1/1
  In1/1 -> Dead Zone/1
  Dead Zone/1 -> P/1, Derivative/1

== system salpChain17/Middle Salp Odd/2DOFJointConstrainer/AnglleConstrainer2 ==
  In1 : Inport
  Dead Zone : DeadZone  LowerValue=-angleLimit  UpperValue=angleLimit  LinearizeAsGain=off  SaturateOnIntegerOverflow=on
  Derivative : Derivative
  P : Gain  Gain=-angleConstraintK
  P1 : Gain  Gain=-angleConstraintB
  Sum : Sum  Inputs=|++
  Out1 : Outport
  wires:
  Derivative/1 -> P1/1
  P1/1 -> Sum/2
  P/1 -> Sum/1
  Sum/1 -> Out1/1
  In1/1 -> Dead Zone/1
  Dead Zone/1 -> P/1, Derivative/1

== system salpChain17/Salp Even/2DOFJointConstrainer/AnglleConstrainer1 ==
  In1 : Inport
  Dead Zone : DeadZone  LowerValue=-angleLimit  UpperValue=angleLimit  LinearizeAsGain=off  SaturateOnIntegerOverflow=on
  Derivative : Derivative
  P : Gain  Gain=-angleConstraintK
  P1 : Gain  Gain=-angleConstraintB
  Sum : Sum  Inputs=|++
  Out1 : Outport
  wires:
  Derivative/1 -> P1/1
  P1/1 -> Sum/2
  P/1 -> Sum/1
  Sum/1 -> Out1/1
  In1/1 -> Dead Zone/1
  Dead Zone/1 -> P/1, Derivative/1

== system salpChain17/Salp Even/2DOFJointConstrainer/AnglleConstrainer2 ==
  In1 : Inport
  Dead Zone : DeadZone  LowerValue=-angleLimit  UpperValue=angleLimit  LinearizeAsGain=off  SaturateOnIntegerOverflow=on
  Derivative : Derivative
  P : Gain  Gain=-angleConstraintK
  P1 : Gain  Gain=-angleConstraintB
  Sum : Sum  Inputs=|++
  Out1 : Outport
  wires:
  Derivative/1 -> P1/1
  P1/1 -> Sum/2
  P/1 -> Sum/1
  Sum/1 -> Out1/1
  In1/1 -> Dead Zone/1
  Dead Zone/1 -> P/1, Derivative/1

== system salpChain17/Salp Even1/2DOFJointConstrainer/AnglleConstrainer1 ==
  In1 : Inport
  Dead Zone : DeadZone  LowerValue=-angleLimit  UpperValue=angleLimit  LinearizeAsGain=off  SaturateOnIntegerOverflow=on
  Derivative : Derivative
  P : Gain  Gain=-angleConstraintK
  P1 : Gain  Gain=-angleConstraintB
  Sum : Sum  Inputs=|++
  Out1 : Outport
  wires:
  Derivative/1 -> P1/1
  P1/1 -> Sum/2
  P/1 -> Sum/1
  Sum/1 -> Out1/1
  In1/1 -> Dead Zone/1
  Dead Zone/1 -> P/1, Derivative/1

== system salpChain17/Salp Even1/2DOFJointConstrainer/AnglleConstrainer2 ==
  In1 : Inport
  Dead Zone : DeadZone  LowerValue=-angleLimit  UpperValue=angleLimit  LinearizeAsGain=off  SaturateOnIntegerOverflow=on
  Derivative : Derivative
  P : Gain  Gain=-angleConstraintK
  P1 : Gain  Gain=-angleConstraintB
  Sum : Sum  Inputs=|++
  Out1 : Outport
  wires:
  Derivative/1 -> P1/1
  P1/1 -> Sum/2
  P/1 -> Sum/1
  Sum/1 -> Out1/1
  In1/1 -> Dead Zone/1
  Dead Zone/1 -> P/1, Derivative/1

== system salpChain17/Salp Even2/2DOFJointConstrainer/AnglleConstrainer1 ==
  In1 : Inport
  Dead Zone : DeadZone  LowerValue=-angleLimit  UpperValue=angleLimit  LinearizeAsGain=off  SaturateOnIntegerOverflow=on
  Derivative : Derivative
  P : Gain  Gain=-angleConstraintK
  P1 : Gain  Gain=-angleConstraintB
  Sum : Sum  Inputs=|++
  Out1 : Outport
  wires:
  Derivative/1 -> P1/1
  P1/1 -> Sum/2
  P/1 -> Sum/1
  Sum/1 -> Out1/1
  In1/1 -> Dead Zone/1
  Dead Zone/1 -> P/1, Derivative/1

== system salpChain17/Salp Even2/2DOFJointConstrainer/AnglleConstrainer2 ==
  In1 : Inport
  Dead Zone : DeadZone  LowerValue=-angleLimit  UpperValue=angleLimit  LinearizeAsGain=off  SaturateOnIntegerOverflow=on
  Derivative : Derivative
  P : Gain  Gain=-angleConstraintK
  P1 : Gain  Gain=-angleConstraintB
  Sum : Sum  Inputs=|++
  Out1 : Outport
  wires:
  Derivative/1 -> P1/1
  P1/1 -> Sum/2
  P/1 -> Sum/1
  Sum/1 -> Out1/1
  In1/1 -> Dead Zone/1
  Dead Zone/1 -> P/1, Derivative/1

== system salpChain17/Salp Even3/2DOFJointConstrainer/AnglleConstrainer1 ==
  In1 : Inport
  Dead Zone : DeadZone  LowerValue=-angleLimit  UpperValue=angleLimit  LinearizeAsGain=off  SaturateOnIntegerOverflow=on
  Derivative : Derivative
  P : Gain  Gain=-angleConstraintK
  P1 : Gain  Gain=-angleConstraintB
  Sum : Sum  Inputs=|++
  Out1 : Outport
  wires:
  Derivative/1 -> P1/1
  P1/1 -> Sum/2
  P/1 -> Sum/1
  Sum/1 -> Out1/1
  In1/1 -> Dead Zone/1
  Dead Zone/1 -> P/1, Derivative/1

== system salpChain17/Salp Even3/2DOFJointConstrainer/AnglleConstrainer2 ==
  In1 : Inport
  Dead Zone : DeadZone  LowerValue=-angleLimit  UpperValue=angleLimit  LinearizeAsGain=off  SaturateOnIntegerOverflow=on
  Derivative : Derivative
  P : Gain  Gain=-angleConstraintK
  P1 : Gain  Gain=-angleConstraintB
  Sum : Sum  Inputs=|++
  Out1 : Outport
  wires:
  Derivative/1 -> P1/1
  P1/1 -> Sum/2
  P/1 -> Sum/1
  Sum/1 -> Out1/1
  In1/1 -> Dead Zone/1
  Dead Zone/1 -> P/1, Derivative/1

== system salpChain17/Salp Even4/2DOFJointConstrainer/AnglleConstrainer1 ==
  In1 : Inport
  Dead Zone : DeadZone  LowerValue=-angleLimit  UpperValue=angleLimit  LinearizeAsGain=off  SaturateOnIntegerOverflow=on
  Derivative : Derivative
  P : Gain  Gain=-angleConstraintK
  P1 : Gain  Gain=-angleConstraintB
  Sum : Sum  Inputs=|++
  Out1 : Outport
  wires:
  Derivative/1 -> P1/1
  P1/1 -> Sum/2
  P/1 -> Sum/1
  Sum/1 -> Out1/1
  In1/1 -> Dead Zone/1
  Dead Zone/1 -> P/1, Derivative/1

== system salpChain17/Salp Even4/2DOFJointConstrainer/AnglleConstrainer2 ==
  In1 : Inport
  Dead Zone : DeadZone  LowerValue=-angleLimit  UpperValue=angleLimit  LinearizeAsGain=off  SaturateOnIntegerOverflow=on
  Derivative : Derivative
  P : Gain  Gain=-angleConstraintK
  P1 : Gain  Gain=-angleConstraintB
  Sum : Sum  Inputs=|++
  Out1 : Outport
  wires:
  Derivative/1 -> P1/1
  P1/1 -> Sum/2
  P/1 -> Sum/1
  Sum/1 -> Out1/1
  In1/1 -> Dead Zone/1
  Dead Zone/1 -> P/1, Derivative/1

== system salpChain17/Salp Even5/2DOFJointConstrainer/AnglleConstrainer1 ==
  In1 : Inport
  Dead Zone : DeadZone  LowerValue=-angleLimit  UpperValue=angleLimit  LinearizeAsGain=off  SaturateOnIntegerOverflow=on
  Derivative : Derivative
  P : Gain  Gain=-angleConstraintK
  P1 : Gain  Gain=-angleConstraintB
  Sum : Sum  Inputs=|++
  Out1 : Outport
  wires:
  Derivative/1 -> P1/1
  P1/1 -> Sum/2
  P/1 -> Sum/1
  Sum/1 -> Out1/1
  In1/1 -> Dead Zone/1
  Dead Zone/1 -> P/1, Derivative/1

== system salpChain17/Salp Even5/2DOFJointConstrainer/AnglleConstrainer2 ==
  In1 : Inport
  Dead Zone : DeadZone  LowerValue=-angleLimit  UpperValue=angleLimit  LinearizeAsGain=off  SaturateOnIntegerOverflow=on
  Derivative : Derivative
  P : Gain  Gain=-angleConstraintK
  P1 : Gain  Gain=-angleConstraintB
  Sum : Sum  Inputs=|++
  Out1 : Outport
  wires:
  Derivative/1 -> P1/1
  P1/1 -> Sum/2
  P/1 -> Sum/1
  Sum/1 -> Out1/1
  In1/1 -> Dead Zone/1
  Dead Zone/1 -> P/1, Derivative/1

== system salpChain17/Salp Even6/2DOFJointConstrainer/AnglleConstrainer1 ==
  In1 : Inport
  Dead Zone : DeadZone  LowerValue=-angleLimit  UpperValue=angleLimit  LinearizeAsGain=off  SaturateOnIntegerOverflow=on
  Derivative : Derivative
  P : Gain  Gain=-angleConstraintK
  P1 : Gain  Gain=-angleConstraintB
  Sum : Sum  Inputs=|++
  Out1 : Outport
  wires:
  Derivative/1 -> P1/1
  P1/1 -> Sum/2
  P/1 -> Sum/1
  Sum/1 -> Out1/1
  In1/1 -> Dead Zone/1
  Dead Zone/1 -> P/1, Derivative/1

== system salpChain17/Salp Even6/2DOFJointConstrainer/AnglleConstrainer2 ==
  In1 : Inport
  Dead Zone : DeadZone  LowerValue=-angleLimit  UpperValue=angleLimit  LinearizeAsGain=off  SaturateOnIntegerOverflow=on
  Derivative : Derivative
  P : Gain  Gain=-angleConstraintK
  P1 : Gain  Gain=-angleConstraintB
  Sum : Sum  Inputs=|++
  Out1 : Outport
  wires:
  Derivative/1 -> P1/1
  P1/1 -> Sum/2
  P/1 -> Sum/1
  Sum/1 -> Out1/1
  In1/1 -> Dead Zone/1
  Dead Zone/1 -> P/1, Derivative/1

== system salpChain17/Salp Odd/2DOFJointConstrainer/AnglleConstrainer1 ==
  In1 : Inport
  Dead Zone : DeadZone  LowerValue=-angleLimit  UpperValue=angleLimit  LinearizeAsGain=off  SaturateOnIntegerOverflow=on
  Derivative : Derivative
  P : Gain  Gain=-angleConstraintK
  P1 : Gain  Gain=-angleConstraintB
  Sum : Sum  Inputs=|++
  Out1 : Outport
  wires:
  Derivative/1 -> P1/1
  P1/1 -> Sum/2
  P/1 -> Sum/1
  Sum/1 -> Out1/1
  In1/1 -> Dead Zone/1
  Dead Zone/1 -> P/1, Derivative/1

== system salpChain17/Salp Odd/2DOFJointConstrainer/AnglleConstrainer2 ==
  In1 : Inport
  Dead Zone : DeadZone  LowerValue=-angleLimit  UpperValue=angleLimit  LinearizeAsGain=off  SaturateOnIntegerOverflow=on
  Derivative : Derivative
  P : Gain  Gain=-angleConstraintK
  P1 : Gain  Gain=-angleConstraintB
  Sum : Sum  Inputs=|++
  Out1 : Outport
  wires:
  Derivative/1 -> P1/1
  P1/1 -> Sum/2
  P/1 -> Sum/1
  Sum/1 -> Out1/1
  In1/1 -> Dead Zone/1
  Dead Zone/1 -> P/1, Derivative/1

== system salpChain17/Salp Odd1/2DOFJointConstrainer/AnglleConstrainer1 ==
  In1 : Inport
  Dead Zone : DeadZone  LowerValue=-angleLimit  UpperValue=angleLimit  LinearizeAsGain=off  SaturateOnIntegerOverflow=on
  Derivative : Derivative
  P : Gain  Gain=-angleConstraintK
  P1 : Gain  Gain=-angleConstraintB
  Sum : Sum  Inputs=|++
  Out1 : Outport
  wires:
  Derivative/1 -> P1/1
  P1/1 -> Sum/2
  P/1 -> Sum/1
  Sum/1 -> Out1/1
  In1/1 -> Dead Zone/1
  Dead Zone/1 -> P/1, Derivative/1

== system salpChain17/Salp Odd1/2DOFJointConstrainer/AnglleConstrainer2 ==
  In1 : Inport
  Dead Zone : DeadZone  LowerValue=-angleLimit  UpperValue=angleLimit  LinearizeAsGain=off  SaturateOnIntegerOverflow=on
  Derivative : Derivative
  P : Gain  Gain=-angleConstraintK
  P1 : Gain  Gain=-angleConstraintB
  Sum : Sum  Inputs=|++
  Out1 : Outport
  wires:
  Derivative/1 -> P1/1
  P1/1 -> Sum/2
  P/1 -> Sum/1
  Sum/1 -> Out1/1
  In1/1 -> Dead Zone/1
  Dead Zone/1 -> P/1, Derivative/1

== system salpChain17/Salp Odd2/2DOFJointConstrainer/AnglleConstrainer1 ==
  In1 : Inport
  Dead Zone : DeadZone  LowerValue=-angleLimit  UpperValue=angleLimit  LinearizeAsGain=off  SaturateOnIntegerOverflow=on
  Derivative : Derivative
  P : Gain  Gain=-angleConstraintK
  P1 : Gain  Gain=-angleConstraintB
  Sum : Sum  Inputs=|++
  Out1 : Outport
  wires:
  Derivative/1 -> P1/1
  P1/1 -> Sum/2
  P/1 -> Sum/1
  Sum/1 -> Out1/1
  In1/1 -> Dead Zone/1
  Dead Zone/1 -> P/1, Derivative/1

== system salpChain17/Salp Odd2/2DOFJointConstrainer/AnglleConstrainer2 ==
  In1 : Inport
  Dead Zone : DeadZone  LowerValue=-angleLimit  UpperValue=angleLimit  LinearizeAsGain=off  SaturateOnIntegerOverflow=on
  Derivative : Derivative
  P : Gain  Gain=-angleConstraintK
  P1 : Gain  Gain=-angleConstraintB
  Sum : Sum  Inputs=|++
  Out1 : Outport
  wires:
  Derivative/1 -> P1/1
  P1/1 -> Sum/2
  P/1 -> Sum/1
  Sum/1 -> Out1/1
  In1/1 -> Dead Zone/1
  Dead Zone/1 -> P/1, Derivative/1

== system salpChain17/Salp Odd3/2DOFJointConstrainer/AnglleConstrainer1 ==
  In1 : Inport
  Dead Zone : DeadZone  LowerValue=-angleLimit  UpperValue=angleLimit  LinearizeAsGain=off  SaturateOnIntegerOverflow=on
  Derivative : Derivative
  P : Gain  Gain=-angleConstraintK
  P1 : Gain  Gain=-angleConstraintB
  Sum : Sum  Inputs=|++
  Out1 : Outport
  wires:
  Derivative/1 -> P1/1
  P1/1 -> Sum/2
  P/1 -> Sum/1
  Sum/1 -> Out1/1
  In1/1 -> Dead Zone/1
  Dead Zone/1 -> P/1, Derivative/1

== system salpChain17/Salp Odd3/2DOFJointConstrainer/AnglleConstrainer2 ==
  In1 : Inport
  Dead Zone : DeadZone  LowerValue=-angleLimit  UpperValue=angleLimit  LinearizeAsGain=off  SaturateOnIntegerOverflow=on
  Derivative : Derivative
  P : Gain  Gain=-angleConstraintK
  P1 : Gain  Gain=-angleConstraintB
  Sum : Sum  Inputs=|++
  Out1 : Outport
  wires:
  Derivative/1 -> P1/1
  P1/1 -> Sum/2
  P/1 -> Sum/1
  Sum/1 -> Out1/1
  In1/1 -> Dead Zone/1
  Dead Zone/1 -> P/1, Derivative/1

== system salpChain17/Salp Odd4/2DOFJointConstrainer/AnglleConstrainer1 ==
  In1 : Inport
  Dead Zone : DeadZone  LowerValue=-angleLimit  UpperValue=angleLimit  LinearizeAsGain=off  SaturateOnIntegerOverflow=on
  Derivative : Derivative
  P : Gain  Gain=-angleConstraintK
  P1 : Gain  Gain=-angleConstraintB
  Sum : Sum  Inputs=|++
  Out1 : Outport
  wires:
  Derivative/1 -> P1/1
  P1/1 -> Sum/2
  P/1 -> Sum/1
  Sum/1 -> Out1/1
  In1/1 -> Dead Zone/1
  Dead Zone/1 -> P/1, Derivative/1

== system salpChain17/Salp Odd4/2DOFJointConstrainer/AnglleConstrainer2 ==
  In1 : Inport
  Dead Zone : DeadZone  LowerValue=-angleLimit  UpperValue=angleLimit  LinearizeAsGain=off  SaturateOnIntegerOverflow=on
  Derivative : Derivative
  P : Gain  Gain=-angleConstraintK
  P1 : Gain  Gain=-angleConstraintB
  Sum : Sum  Inputs=|++
  Out1 : Outport
  wires:
  Derivative/1 -> P1/1
  P1/1 -> Sum/2
  P/1 -> Sum/1
  Sum/1 -> Out1/1
  In1/1 -> Dead Zone/1
  Dead Zone/1 -> P/1, Derivative/1

== system salpChain17/Salp Odd5/2DOFJointConstrainer/AnglleConstrainer1 ==
  In1 : Inport
  Dead Zone : DeadZone  LowerValue=-angleLimit  UpperValue=angleLimit  LinearizeAsGain=off  SaturateOnIntegerOverflow=on
  Derivative : Derivative
  P : Gain  Gain=-angleConstraintK
  P1 : Gain  Gain=-angleConstraintB
  Sum : Sum  Inputs=|++
  Out1 : Outport
  wires:
  Derivative/1 -> P1/1
  P1/1 -> Sum/2
  P/1 -> Sum/1
  Sum/1 -> Out1/1
  In1/1 -> Dead Zone/1
  Dead Zone/1 -> P/1, Derivative/1

== system salpChain17/Salp Odd5/2DOFJointConstrainer/AnglleConstrainer2 ==
  In1 : Inport
  Dead Zone : DeadZone  LowerValue=-angleLimit  UpperValue=angleLimit  LinearizeAsGain=off  SaturateOnIntegerOverflow=on
  Derivative : Derivative
  P : Gain  Gain=-angleConstraintK
  P1 : Gain  Gain=-angleConstraintB
  Sum : Sum  Inputs=|++
  Out1 : Outport
  wires:
  Derivative/1 -> P1/1
  P1/1 -> Sum/2
  P/1 -> Sum/1
  Sum/1 -> Out1/1
  In1/1 -> Dead Zone/1
  Dead Zone/1 -> P/1, Derivative/1

== system salpChain17/preEnd Salp Even/2DOFJointConstrainer/AnglleConstrainer1 ==
  In1 : Inport
  Dead Zone : DeadZone  LowerValue=-angleLimit  UpperValue=angleLimit  LinearizeAsGain=off  SaturateOnIntegerOverflow=on
  Derivative : Derivative
  P : Gain  Gain=-angleConstraintK
  P1 : Gain  Gain=-angleConstraintB
  Sum : Sum  Inputs=|++
  Out1 : Outport
  wires:
  Derivative/1 -> P1/1
  P1/1 -> Sum/2
  P/1 -> Sum/1
  Sum/1 -> Out1/1
  In1/1 -> Dead Zone/1
  Dead Zone/1 -> P/1, Derivative/1

== system salpChain17/preEnd Salp Even/2DOFJointConstrainer/AnglleConstrainer2 ==
  In1 : Inport
  Dead Zone : DeadZone  LowerValue=-angleLimit  UpperValue=angleLimit  LinearizeAsGain=off  SaturateOnIntegerOverflow=on
  Derivative : Derivative
  P : Gain  Gain=-angleConstraintK
  P1 : Gain  Gain=-angleConstraintB
  Sum : Sum  Inputs=|++
  Out1 : Outport
  wires:
  Derivative/1 -> P1/1
  P1/1 -> Sum/2
  P/1 -> Sum/1
  Sum/1 -> Out1/1
  In1/1 -> Dead Zone/1
  Dead Zone/1 -> P/1, Derivative/1
